simulink model "HMIHeightSelc"  (R2018b)
settings: Solver=FixedStepDiscrete  StartTime=0.0  StopTime=10.0  FixedStep=0.01  RelTol=1e-3
undefined symbols (not defined in the file or in its folder): arg, EEPHMISecRwStPassHeight_Set, KeSMSeHeiCstTypeConfig_Val
settings Model: Creator=sn2xws  LastModifiedBy=sn2xws
settings DataIOCC: SaveFormat=StructureWithTime
settings OptimizationCC: DefaultParameterBehavior=Inlined  EnhancedBackFolding=on  PassReuseOutputArgsAs=Individual arguments  ZeroExternalMemoryAtStartup=off  ZeroInternalMemoryAtStartup=off  OptimizeBlockOrder=speed  DifferentSizesBufferReuse=on  OptimizationCustomize=off
settings DebuggingCC: ParameterTunabilityLossMsg=error
settings ModelReferenceCC: ModelReferenceNumInstancesAllowed=Single
settings SFSimCC: MATLABDynamicMemAlloc=off
settings RTWCC: SystemTargetFile=autosar.tlc  GenCodeOnly=on  TemplateMakefile=ert_default_tmf  Description=AUTOSAR  GenerateReport=on  IncludeHyperlinkInReport=on  LaunchReport=on  GenerateTraceInfo=on  GenerateTraceReport=on  GenerateTraceReportSl=on  GenerateTraceReportSf=on  GenerateTraceReportEml=on  GenerateCodeMetricsReport=on
settings CodeAppCC: ForceParamTrailComments=on  IgnoreCustomStorageClasses=off  OperatorAnnotations=on  SimulinkDataObjDesc=on  SFDataObjDesc=on  InsertBlockDesc=on
settings STFCustomTargetCC: TargetLangStandard=C99 (ISO)  MultiwordLength=256  ParMdlRefBuildCompliant=on  CompOptLevelCompliant=on  IncludeMdlTerminateFcn=off  CombineOutputUpdateFcns=on  SuppressErrorStatus=on  ERTCustomFileBanners=on  SupportNonFinite=off  SupportComplex=off  SupportContinuousTime=off  SupportNonInlinedSFcns=off  RemoveResetFunc=on  MATLABClassNameForMDSCustomization=Simulink.SoftwareTarget.ERTCustomization  AutosarCompliant=on  UseToolchainInfoCompliant=on  LookupTableObjectStructAxisOrder=2,1,3,4,...  LUTObjectStructOrderEvenSpacing=Size,Table,Breakpoints  SystemTargetFile=autosar.tlc
settings ERTTargetCC: TargetLangStandard=C99 (ISO)  ConcurrentExecutionCompliant=off  IncludeMdlTerminateFcn=off  SuppressErrorStatus=on  SupportNonFinite=off  SupportComplex=off  ModelStepFunctionPrototypeControlCompliant=off  CPPClassGenCompliant=off  AutosarCompliant=on  LookupTableObjectStructAxisOrder=2,1,3,4,...  LUTObjectStructOrderEvenSpacing=Size,Table,Breakpoints  InlinedParameterPlacement=NonHierarchical  ERTCustomFileTemplate=example_file_process.tlc

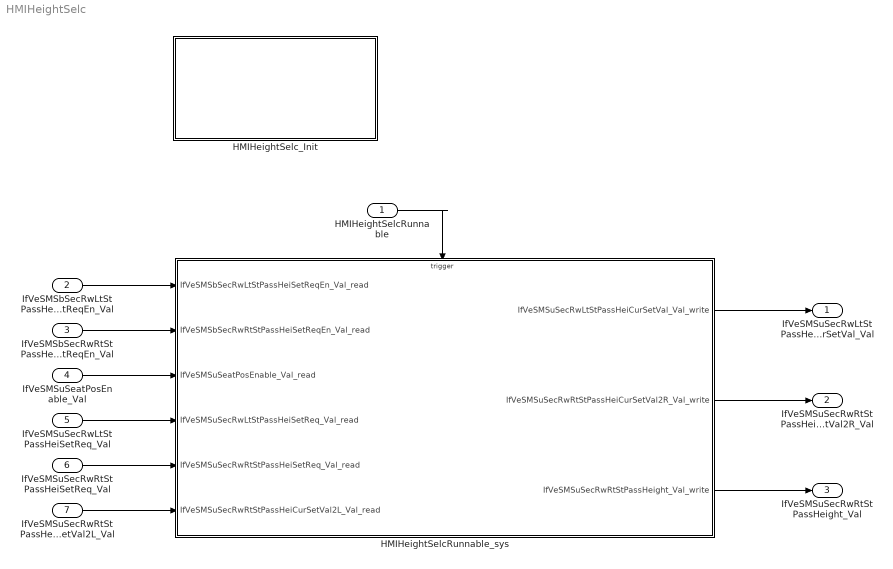
== system HMIHeightSelc ==
  HMIHeightSelcRunnable : Inport  SampleTime=0.01  OutputFunctionCall=on
  IfVeSMSbSecRwLtStPassHeiSetReqEn_Val : Inport  Port=2  OutDataTypeStr=boolean  PortDimensions=1
  IfVeSMSbSecRwRtStPassHeiSetReqEn_Val : Inport  Port=3  OutDataTypeStr=boolean  PortDimensions=1
  IfVeSMSuSeatPosEnable_Val : Inport  Port=4  OutDataTypeStr=uint8  PortDimensions=1
  IfVeSMSuSecRwLtStPassHeiSetReq_Val : Inport  Port=5  OutDataTypeStr=uint8  PortDimensions=1
  IfVeSMSuSecRwRtStPassHeiSetReq_Val : Inport  Port=6  OutDataTypeStr=uint8  PortDimensions=1
  IfVeSMSuSecRwRtStPassHeiCurSetVal2L_Val : Inport  Port=7  OutDataTypeStr=uint8  PortDimensions=1
  HMIHeightSelcRunnable_sys : Subsystem
  HMIHeightSelc_Init : Subsystem
  IfVeSMSuSecRwLtStPassHeiCurSetVal_Val : Outport  OutDataTypeStr=uint8  PortDimensions=1
  IfVeSMSuSecRwRtStPassHeiCurSetVal2R_Val : Outport  Port=2  OutDataTypeStr=uint8  PortDimensions=1
  IfVeSMSuSecRwRtStPassHeight_Val : Outport  Port=3  OutDataTypeStr=uint8  PortDimensions=1
  wires:
  IfVeSMSbSecRwLtStPassHeiSetReqEn_Val/1 -> HMIHeightSelcRunnable_sys/1(IfVeSMSbSecRwLtStPassHeiSetReqEn_Val_read)
  IfVeSMSbSecRwRtStPassHeiSetReqEn_Val/1 -> HMIHeightSelcRunnable_sys/2(IfVeSMSbSecRwRtStPassHeiSetReqEn_Val_read)
  IfVeSMSuSeatPosEnable_Val/1 -> HMIHeightSelcRunnable_sys/3(IfVeSMSuSeatPosEnable_Val_read)
  IfVeSMSuSecRwLtStPassHeiSetReq_Val/1 -> HMIHeightSelcRunnable_sys/4(IfVeSMSuSecRwLtStPassHeiSetReq_Val_read)
  IfVeSMSuSecRwRtStPassHeiSetReq_Val/1 -> HMIHeightSelcRunnable_sys/5(IfVeSMSuSecRwRtStPassHeiSetReq_Val_read)
  IfVeSMSuSecRwRtStPassHeiCurSetVal2L_Val/1 -> HMIHeightSelcRunnable_sys/6(IfVeSMSuSecRwRtStPassHeiCurSetVal2L_Val_read)
  HMIHeightSelcRunnable_sys/1(IfVeSMSuSecRwLtStPassHeiCurSetVal_Val_write) -> IfVeSMSuSecRwLtStPassHeiCurSetVal_Val/1
  HMIHeightSelcRunnable_sys/2(IfVeSMSuSecRwRtStPassHeiCurSetVal2R_Val_write) -> IfVeSMSuSecRwRtStPassHeiCurSetVal2R_Val/1
  HMIHeightSelcRunnable_sys/3(IfVeSMSuSecRwRtStPassHeight_Val_write) -> IfVeSMSuSecRwRtStPassHeight_Val/1
  HMIHeightSelcRunnable/1 -> HMIHeightSelcRunnable_sys/Trigger

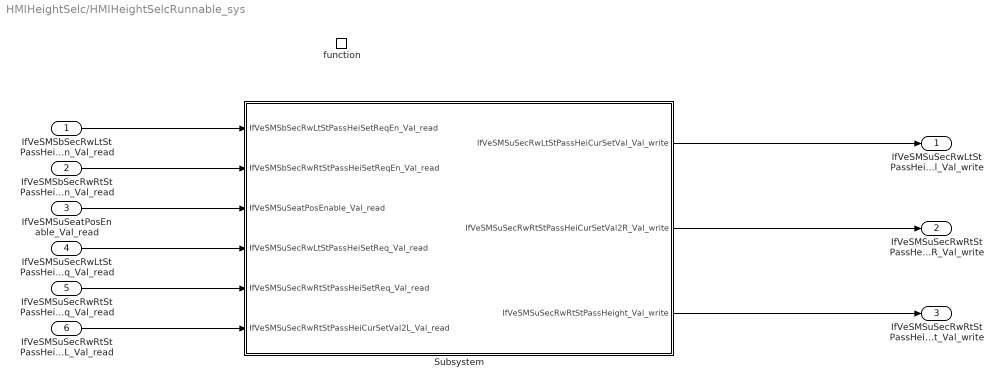
== system HMIHeightSelc/HMIHeightSelcRunnable_sys ==
  IfVeSMSbSecRwLtStPassHeiSetReqEn_Val_read : Inport
  IfVeSMSbSecRwRtStPassHeiSetReqEn_Val_read : Inport  Port=2
  IfVeSMSuSeatPosEnable_Val_read : Inport  Port=3
  IfVeSMSuSecRwLtStPassHeiSetReq_Val_read : Inport  Port=4
  IfVeSMSuSecRwRtStPassHeiSetReq_Val_read : Inport  Port=5
  IfVeSMSuSecRwRtStPassHeiCurSetVal2L_Val_read : Inport  Port=6
  function : TriggerPort  TriggerType=function-call  VariantControl=(inherit)  SampleTimeType=periodic  SampleTime=-1
  Subsystem : Subsystem
  IfVeSMSuSecRwLtStPassHeiCurSetVal_Val_write : Outport
      settings: EnsureOutportIsVirtual=on
  IfVeSMSuSecRwRtStPassHeiCurSetVal2R_Val_write : Outport  Port=2
      settings: EnsureOutportIsVirtual=on
  IfVeSMSuSecRwRtStPassHeight_Val_write : Outport  Port=3
      settings: EnsureOutportIsVirtual=on
  wires:
  IfVeSMSbSecRwLtStPassHeiSetReqEn_Val_read/1 -> Subsystem/1(IfVeSMSbSecRwLtStPassHeiSetReqEn_Val_read)
  IfVeSMSbSecRwRtStPassHeiSetReqEn_Val_read/1 -> Subsystem/2(IfVeSMSbSecRwRtStPassHeiSetReqEn_Val_read)
  IfVeSMSuSeatPosEnable_Val_read/1 -> Subsystem/3(IfVeSMSuSeatPosEnable_Val_read)
  IfVeSMSuSecRwLtStPassHeiSetReq_Val_read/1 -> Subsystem/4(IfVeSMSuSecRwLtStPassHeiSetReq_Val_read)
  IfVeSMSuSecRwRtStPassHeiSetReq_Val_read/1 -> Subsystem/5(IfVeSMSuSecRwRtStPassHeiSetReq_Val_read)
  IfVeSMSuSecRwRtStPassHeiCurSetVal2L_Val_read/1 -> Subsystem/6(IfVeSMSuSecRwRtStPassHeiCurSetVal2L_Val_read)
  Subsystem/1(IfVeSMSuSecRwLtStPassHeiCurSetVal_Val_write) -> IfVeSMSuSecRwLtStPassHeiCurSetVal_Val_write/1
  Subsystem/2(IfVeSMSuSecRwRtStPassHeiCurSetVal2R_Val_write) -> IfVeSMSuSecRwRtStPassHeiCurSetVal2R_Val_write/1
  Subsystem/3(IfVeSMSuSecRwRtStPassHeight_Val_write) -> IfVeSMSuSecRwRtStPassHeight_Val_write/1

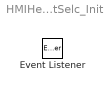
== system HMIHeightSelc/HMIHeightSelc_Init ==
  Event Listener : EventListener  EventName=reset

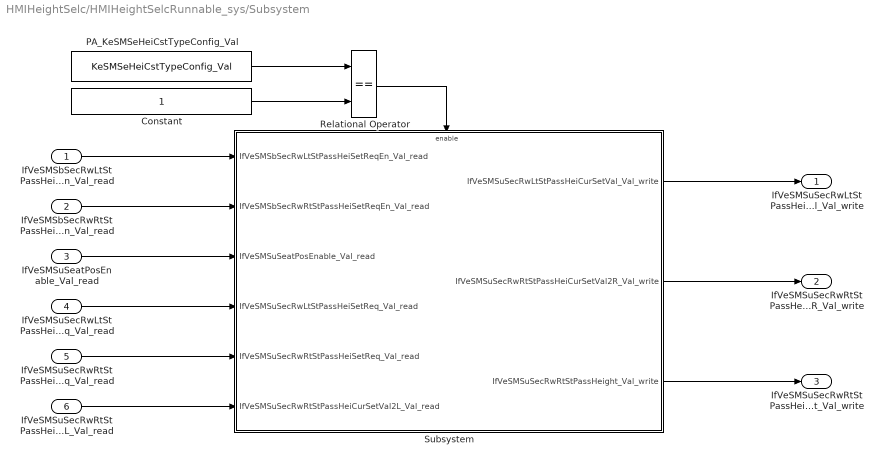
== system HMIHeightSelc/HMIHeightSelcRunnable_sys/Subsystem ==
  IfVeSMSbSecRwLtStPassHeiSetReqEn_Val_read : Inport
  IfVeSMSbSecRwRtStPassHeiSetReqEn_Val_read : Inport  Port=2
  IfVeSMSuSeatPosEnable_Val_read : Inport  Port=3
  IfVeSMSuSecRwLtStPassHeiSetReq_Val_read : Inport  Port=4
  IfVeSMSuSecRwRtStPassHeiSetReq_Val_read : Inport  Port=5
  IfVeSMSuSecRwRtStPassHeiCurSetVal2L_Val_read : Inport  Port=6
  Constant : Constant  OutDataTypeStr=uint8
  PA_KeSMSeHeiCstTypeConfig_Val : Constant  Value=KeSMSeHeiCstTypeConfig_Val
  Relational Operator : RelationalOperator  Operator===  OutDataTypeStr=boolean  RndMeth=Simplest
  Subsystem : Subsystem
  IfVeSMSuSecRwLtStPassHeiCurSetVal_Val_write : Outport
      settings: EnsureOutportIsVirtual=on
  IfVeSMSuSecRwRtStPassHeiCurSetVal2R_Val_write : Outport  Port=2
      settings: EnsureOutportIsVirtual=on
  IfVeSMSuSecRwRtStPassHeight_Val_write : Outport  Port=3
      settings: EnsureOutportIsVirtual=on
  wires:
  PA_KeSMSeHeiCstTypeConfig_Val/1 -> Relational Operator/1
  Constant/1 -> Relational Operator/2
  IfVeSMSbSecRwLtStPassHeiSetReqEn_Val_read/1 -> Subsystem/1(IfVeSMSbSecRwLtStPassHeiSetReqEn_Val_read)
  IfVeSMSbSecRwRtStPassHeiSetReqEn_Val_read/1 -> Subsystem/2(IfVeSMSbSecRwRtStPassHeiSetReqEn_Val_read)
  IfVeSMSuSeatPosEnable_Val_read/1 -> Subsystem/3(IfVeSMSuSeatPosEnable_Val_read)
  IfVeSMSuSecRwLtStPassHeiSetReq_Val_read/1 -> Subsystem/4(IfVeSMSuSecRwLtStPassHeiSetReq_Val_read)
  IfVeSMSuSecRwRtStPassHeiSetReq_Val_read/1 -> Subsystem/5(IfVeSMSuSecRwRtStPassHeiSetReq_Val_read)
  IfVeSMSuSecRwRtStPassHeiCurSetVal2L_Val_read/1 -> Subsystem/6(IfVeSMSuSecRwRtStPassHeiCurSetVal2L_Val_read)
  Subsystem/1(IfVeSMSuSecRwLtStPassHeiCurSetVal_Val_write) -> IfVeSMSuSecRwLtStPassHeiCurSetVal_Val_write/1
  Subsystem/2(IfVeSMSuSecRwRtStPassHeiCurSetVal2R_Val_write) -> IfVeSMSuSecRwRtStPassHeiCurSetVal2R_Val_write/1
  Subsystem/3(IfVeSMSuSecRwRtStPassHeight_Val_write) -> IfVeSMSuSecRwRtStPassHeight_Val_write/1
  Relational Operator/1 -> Subsystem/Enable

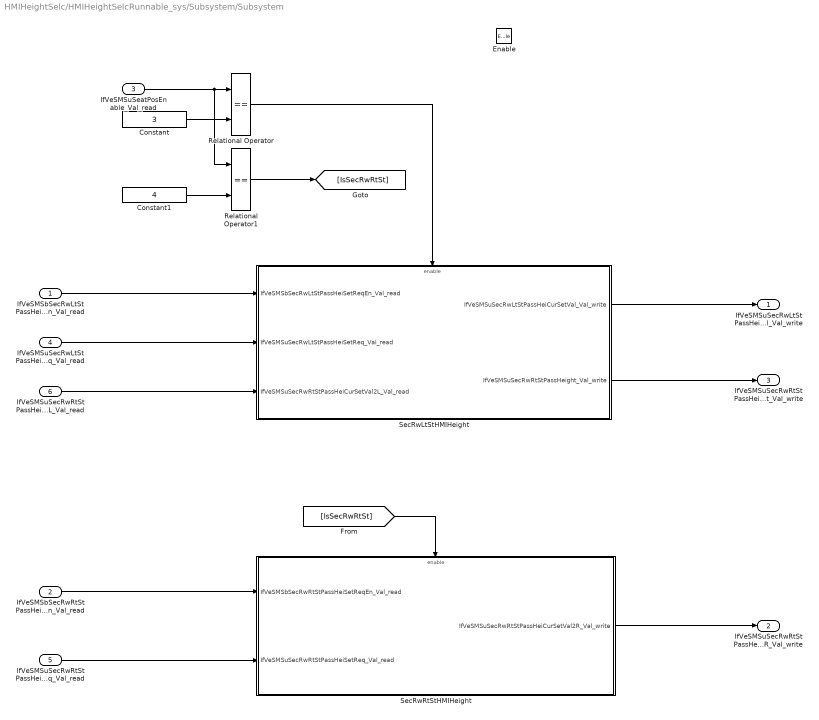
== system HMIHeightSelc/HMIHeightSelcRunnable_sys/Subsystem/Subsystem ==
  IfVeSMSbSecRwLtStPassHeiSetReqEn_Val_read : Inport
  IfVeSMSbSecRwRtStPassHeiSetReqEn_Val_read : Inport  Port=2
  IfVeSMSuSeatPosEnable_Val_read : Inport  Port=3
  IfVeSMSuSecRwLtStPassHeiSetReq_Val_read : Inport  Port=4
  IfVeSMSuSecRwRtStPassHeiSetReq_Val_read : Inport  Port=5
  IfVeSMSuSecRwRtStPassHeiCurSetVal2L_Val_read : Inport  Port=6
  Enable : EnablePort
  Constant : Constant  Value=3  OutDataTypeStr=uint8
  Constant1 : Constant  Value=4  OutDataTypeStr=uint8
  Relational Operator : RelationalOperator  Operator===  OutDataTypeStr=boolean  RndMeth=Simplest
  Relational Operator1 : RelationalOperator  Operator===  OutDataTypeStr=boolean  RndMeth=Simplest
  SecRwLtStHMIHeight : Subsystem
  SecRwRtStHMIHeight : Subsystem
  IfVeSMSuSecRwLtStPassHeiCurSetVal_Val_write : Outport
      settings: EnsureOutportIsVirtual=on
  IfVeSMSuSecRwRtStPassHeiCurSetVal2R_Val_write : Outport  Port=2
      settings: EnsureOutportIsVirtual=on
  IfVeSMSuSecRwRtStPassHeight_Val_write : Outport  Port=3
      settings: EnsureOutportIsVirtual=on
  wires:
  IfVeSMSuSeatPosEnable_Val_read/1 -> Relational Operator1/1, Relational Operator/1
  SecRwRtStHMIHeight/1(IfVeSMSuSecRwRtStPassHeiCurSetVal2R_Val_write) -> IfVeSMSuSecRwRtStPassHeiCurSetVal2R_Val_write/1
  SecRwLtStHMIHeight/1(IfVeSMSuSecRwLtStPassHeiCurSetVal_Val_write) -> IfVeSMSuSecRwLtStPassHeiCurSetVal_Val_write/1
  Constant/1 -> Relational Operator/2
  Relational Operator/1 -> SecRwLtStHMIHeight/Enable
  Constant1/1 -> Relational Operator1/2
  Relational Operator1/1 -> [IsSecRwRtSt]
  [IsSecRwRtSt] -> SecRwRtStHMIHeight/Enable
  IfVeSMSbSecRwLtStPassHeiSetReqEn_Val_read/1 -> SecRwLtStHMIHeight/1(IfVeSMSbSecRwLtStPassHeiSetReqEn_Val_read)
  IfVeSMSuSecRwLtStPassHeiSetReq_Val_read/1 -> SecRwLtStHMIHeight/2(IfVeSMSuSecRwLtStPassHeiSetReq_Val_read)
  IfVeSMSuSecRwRtStPassHeiCurSetVal2L_Val_read/1 -> SecRwLtStHMIHeight/3(IfVeSMSuSecRwRtStPassHeiCurSetVal2L_Val_read)
  SecRwLtStHMIHeight/2(IfVeSMSuSecRwRtStPassHeight_Val_write) -> IfVeSMSuSecRwRtStPassHeight_Val_write/1
  IfVeSMSbSecRwRtStPassHeiSetReqEn_Val_read/1 -> SecRwRtStHMIHeight/1(IfVeSMSbSecRwRtStPassHeiSetReqEn_Val_read)
  IfVeSMSuSecRwRtStPassHeiSetReq_Val_read/1 -> SecRwRtStHMIHeight/2(IfVeSMSuSecRwRtStPassHeiSetReq_Val_read)

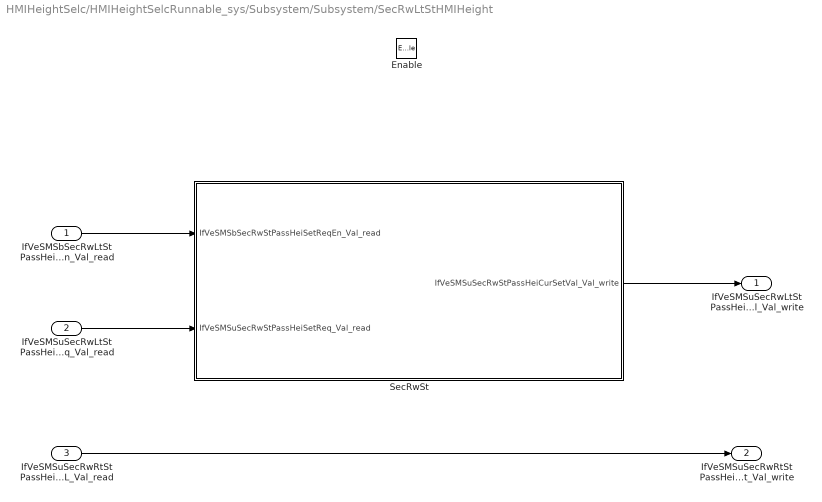
== system HMIHeightSelc/HMIHeightSelcRunnable_sys/Subsystem/Subsystem/SecRwLtStHMIHeight ==
  IfVeSMSbSecRwLtStPassHeiSetReqEn_Val_read : Inport
  IfVeSMSuSecRwLtStPassHeiSetReq_Val_read : Inport  Port=2
  IfVeSMSuSecRwRtStPassHeiCurSetVal2L_Val_read : Inport  Port=3
  Enable : EnablePort
  SecRwSt : Stateflow chart  TreatAsAtomicUnit=on
  IfVeSMSuSecRwLtStPassHeiCurSetVal_Val_write : Outport
      settings: EnsureOutportIsVirtual=on
  IfVeSMSuSecRwRtStPassHeight_Val_write : Outport  Port=2
      settings: EnsureOutportIsVirtual=on
  wires:
  IfVeSMSuSecRwLtStPassHeiSetReq_Val_read/1 -> SecRwSt/2(IfVeSMSuSecRwStPassHeiSetReq_Val_read)
  IfVeSMSuSecRwRtStPassHeiCurSetVal2L_Val_read/1 -> IfVeSMSuSecRwRtStPassHeight_Val_write/1
  IfVeSMSbSecRwLtStPassHeiSetReqEn_Val_read/1 -> SecRwSt/1(IfVeSMSbSecRwStPassHeiSetReqEn_Val_read)
  SecRwSt/1(IfVeSMSuSecRwStPassHeiCurSetVal_Val_write) -> IfVeSMSuSecRwLtStPassHeiCurSetVal_Val_write/1

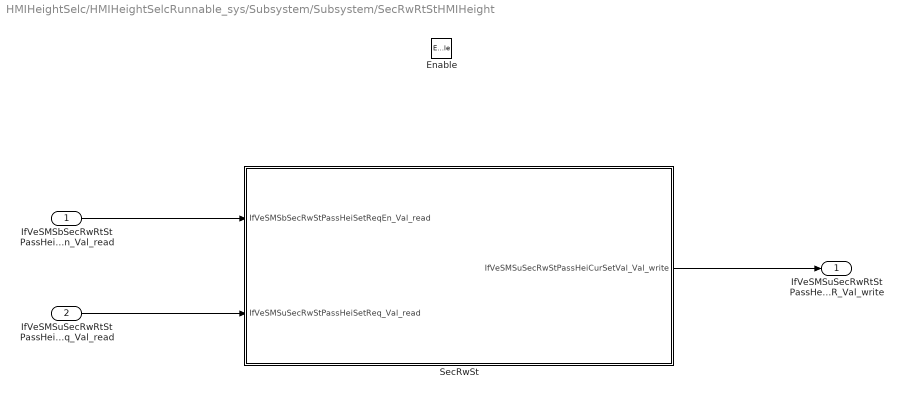
== system HMIHeightSelc/HMIHeightSelcRunnable_sys/Subsystem/Subsystem/SecRwRtStHMIHeight ==
  IfVeSMSbSecRwRtStPassHeiSetReqEn_Val_read : Inport
  IfVeSMSuSecRwRtStPassHeiSetReq_Val_read : Inport  Port=2
  Enable : EnablePort
  SecRwSt : Stateflow chart  TreatAsAtomicUnit=on
  IfVeSMSuSecRwRtStPassHeiCurSetVal2R_Val_write : Outport
      settings: EnsureOutportIsVirtual=on
  wires:
  IfVeSMSbSecRwRtStPassHeiSetReqEn_Val_read/1 -> SecRwSt/1(IfVeSMSbSecRwStPassHeiSetReqEn_Val_read)
  IfVeSMSuSecRwRtStPassHeiSetReq_Val_read/1 -> SecRwSt/2(IfVeSMSuSecRwStPassHeiSetReq_Val_read)
  SecRwSt/1(IfVeSMSuSecRwStPassHeiCurSetVal_Val_write) -> IfVeSMSuSecRwRtStPassHeiCurSetVal2R_Val_write/1

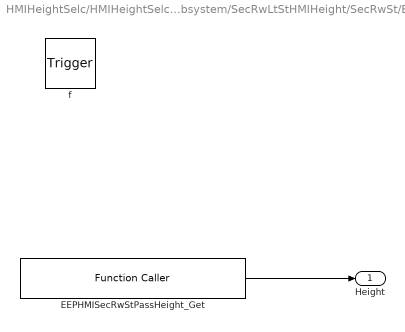
== system HMIHeightSelc/HMIHeightSelcRunnable_sys/Subsystem/Subsystem/SecRwLtStHMIHeight/SecRwSt/EEPHMISecRwStPassHeight_Get ==
  f : TriggerPort  TriggerType=function-call  VariantControl=(inherit)
      settings: CopyFcn=Stateflow.SLINSF.SimulinkMan.removeBlockPreDeleteFcn  PreDeleteFcn=Stateflow.SLINSF.SimulinkMan.unsafePredeleteFcn
  EEPHMISecRwStPassHeight_Get : FunctionCaller  FunctionPrototype=arg = EEPHMISecRwStPassHeight_Get()  OutputArgumentSpecifications=P_EEP_Uint8
  Height : Outport
  wires:
  EEPHMISecRwStPassHeight_Get/1 -> Height/1

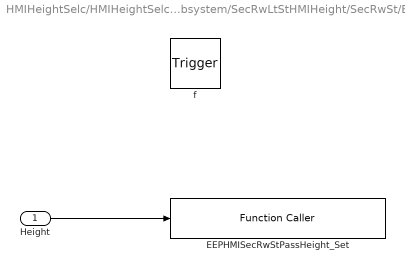
== system HMIHeightSelc/HMIHeightSelcRunnable_sys/Subsystem/Subsystem/SecRwLtStHMIHeight/SecRwSt/EEPHMISecRwStPassHeight_Set ==
  Height : Inport
  f : TriggerPort  TriggerType=function-call  VariantControl=(inherit)
      settings: CopyFcn=Stateflow.SLINSF.SimulinkMan.removeBlockPreDeleteFcn  PreDeleteFcn=Stateflow.SLINSF.SimulinkMan.unsafePredeleteFcn
  EEPHMISecRwStPassHeight_Set : FunctionCaller  FunctionPrototype=EEPHMISecRwStPassHeight_Set(arg)  InputArgumentSpecifications=P_EEP_Uint8
  wires:
  Height/1 -> EEPHMISecRwStPassHeight_Set/1

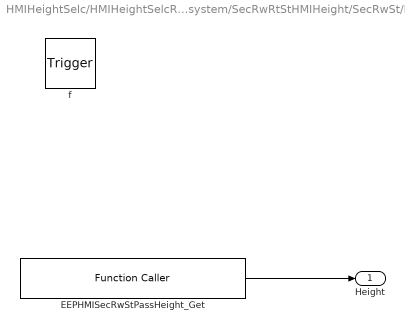
== system HMIHeightSelc/HMIHeightSelcRunnable_sys/Subsystem/Subsystem/SecRwRtStHMIHeight/SecRwSt/EEPHMISecRwStPassHeight_Get ==
  f : TriggerPort  TriggerType=function-call  VariantControl=(inherit)
      settings: CopyFcn=Stateflow.SLINSF.SimulinkMan.removeBlockPreDeleteFcn  PreDeleteFcn=Stateflow.SLINSF.SimulinkMan.unsafePredeleteFcn
  EEPHMISecRwStPassHeight_Get : FunctionCaller  FunctionPrototype=arg = EEPHMISecRwStPassHeight_Get()  OutputArgumentSpecifications=P_EEP_Uint8
  Height : Outport
  wires:
  EEPHMISecRwStPassHeight_Get/1 -> Height/1

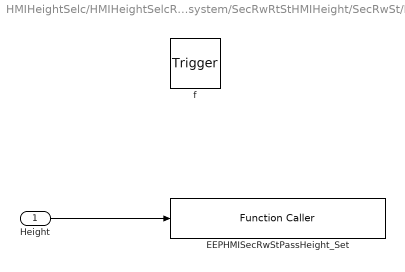
== system HMIHeightSelc/HMIHeightSelcRunnable_sys/Subsystem/Subsystem/SecRwRtStHMIHeight/SecRwSt/EEPHMISecRwStPassHeight_Set ==
  Height : Inport
  f : TriggerPort  TriggerType=function-call  VariantControl=(inherit)
      settings: CopyFcn=Stateflow.SLINSF.SimulinkMan.removeBlockPreDeleteFcn  PreDeleteFcn=Stateflow.SLINSF.SimulinkMan.unsafePredeleteFcn
  EEPHMISecRwStPassHeight_Set : FunctionCaller  FunctionPrototype=EEPHMISecRwStPassHeight_Set(arg)  InputArgumentSpecifications=P_EEP_Uint8
  wires:
  Height/1 -> EEPHMISecRwStPassHeight_Set/1

== stateflow chart HMIHeightSelc/HMIHeightSelcRunnable_sys/Subsystem/Subsystem/SecRwRtStHMIHeight/SecRwSt ==
  state Height =EEPHMISecRwStPassHeight_Get [function]
  state EEPHMISecRwStPassHeight_Set(Height) [function]
  state SecRwSt
    en:IfVeSMSuSecRwStPassHeiCurSetVal_Val_write = LocalHeight;
    du:IfVeSMSuSecRwStPassHeiCurSetVal_Val_write = LocalHeight;
    state HMIConfig
      en:TmpHeight = IfVeSMSuSecRwStPassHeiSetReq_Val_read;
      du:TmpHeight = IfVeSMSuSecRwStPassHeiSetReq_Val_read;
    state ConfirmHeight
      en:LocalHeight = TmpHeight;
      en:EEPHMISecRwStPassHeight_Set(LocalHeight);
    (default) -> ConfirmHeight
    ConfirmHeight -> HMIConfig : [IfVeSMSbSecRwStPassHeiSetReqEn_Val_read]
    HMIConfig -> ConfirmHeight : [!IfVeSMSbSecRwStPassHeiSetReqEn_Val_read]
  (default) -> SecRwSt : {
      | LocalHeight = EEPHMISecRwStPassHeight_Get();
      |  }
  data: Height function_output; Height function_input; IfVeSMSbSecRwStPassHeiSetReqEn_Val_read input; IfVeSMSuSecRwStPassHeiSetReq_Val_read input; IfVeSMSuSecRwStPassHeiCurSetVal_Val_write output; LocalHeight local uint8 =0; TmpHeight local uint8

== stateflow chart HMIHeightSelc/HMIHeightSelcRunnable_sys/Subsystem/Subsystem/SecRwLtStHMIHeight/SecRwSt ==
  state Height =EEPHMISecRwStPassHeight_Get [function]
  state EEPHMISecRwStPassHeight_Set(Height) [function]
  state SecRwSt
    en:IfVeSMSuSecRwStPassHeiCurSetVal_Val_write = LocalHeight;
    du:IfVeSMSuSecRwStPassHeiCurSetVal_Val_write = LocalHeight;
    state HMIConfig
      en:TmpHeight = IfVeSMSuSecRwStPassHeiSetReq_Val_read;
      du:TmpHeight = IfVeSMSuSecRwStPassHeiSetReq_Val_read;
    state ConfirmHeight
      en:LocalHeight = TmpHeight;
      en:EEPHMISecRwStPassHeight_Set(LocalHeight);
    (default) -> ConfirmHeight
    ConfirmHeight -> HMIConfig : [IfVeSMSbSecRwStPassHeiSetReqEn_Val_read]
    HMIConfig -> ConfirmHeight : [!IfVeSMSbSecRwStPassHeiSetReqEn_Val_read]
  (default) -> SecRwSt : {
      | LocalHeight = EEPHMISecRwStPassHeight_Get();
      |  }
  data: Height function_output; Height function_input; IfVeSMSbSecRwStPassHeiSetReqEn_Val_read input; IfVeSMSuSecRwStPassHeiSetReq_Val_read input; IfVeSMSuSecRwStPassHeiCurSetVal_Val_write output; LocalHeight local uint8 =0; TmpHeight local uint8
